simulink model "BPSK____TRANSMITTER"  (R2022a)
settings: Solver=VariableStepAuto  StartTime=0.0  StopTime=inf  RelTol=1e-3
values from neighbouring files (symbols this model uses):
  numSymsTot = length(message)    [generatemessage____BPSK.m]
undefined symbols (not defined in the file or in its folder): Fs, ip, usb
libraries: commfilt2 x2, dspsrcs4 x2, plutoradiolib x1, commdigbbndpm3 x1, simulink x1
settings Model: Creator=Nithish  LastModifiedBy=Nithish

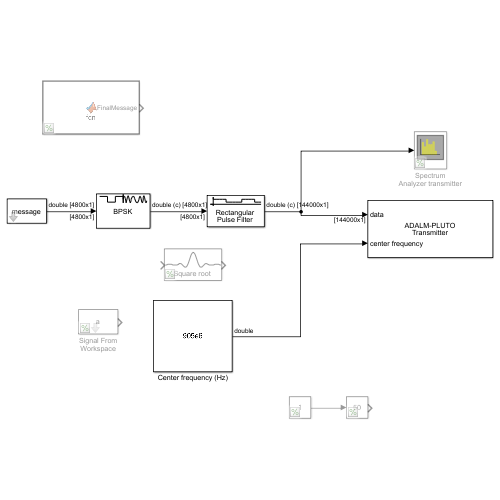
[thumbnail: Simulink's stored preview of the top-level diagram]
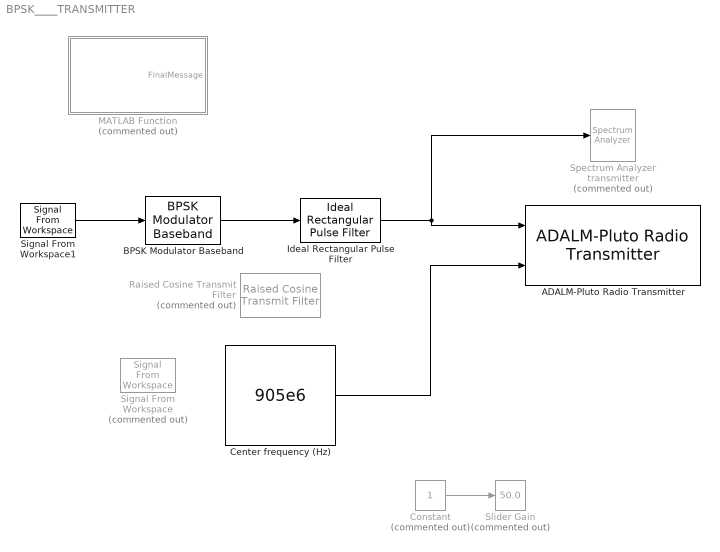
== system BPSK____TRANSMITTER ==
  ADALM-Pluto Radio Transmitter : plutoradiolib/ADALM-Pluto Radio Transmitter  RadioID=usb:0  uri=ip:10.0.0.200  CenterFrequencySource=Input Port  CenterFrequency=2.4e9  GainSource=Dialog  Gain=<binary blob, 139 chars, not shown>  ChannelMapping=1  BasebandSampleRate=240e3  UnderflowOutputPort=off  ShowAdvancedProperties=off  UseCustomFilter=off  filtPathRates=[737280000 11520000 3840000 1920000 960000 240000]  filtCoefficients=[-192 82 85 -215 228 -102 -110 290 -318 145 160 -426 471 -215 -238 633 -697 318 349 -923 1009 -457 -498 1309 -1423 640 693 -1812 1959 -876 -945 2458 -2647 1180 1268 -3290 3534 -1572 -1688 4375 -4698 2091 2247 -5836 6284 -2807 -3031 7918 -8588 3870 4225 -11182 12324 -5662 -6330 17255 -19735 9507 11312 -33568 43355 -25227 -42139 305542 305542 -42139 -25227 43355 -33568 11312 9507 -19735 17255 -6330 -5662 12324 -11182 4225 3870 -8588 7918 -3031 -2807 6284 -5836 2247 2091 -4698 4375 -1688 -1572 3534 -3290 1268 1180 -2647 2458 -945 -876 1959 -1812 693 640 -1423 1309 -498 -457 1009 -923 349 318 -697 633 -238 -215 471 -426 160 145 -318 290 -110 -102 228 -215 85 82 -192]  filtCoefficientSize=128  filtDecimInterpFactor=4  filtGain=-12  filtRFBandwidth=18000000  filterConfigStruct=struct()  DataSourceSelect=Input Port  DDSTone1Freq=5e3  DDSTone2Freq=10e3  DDSTone1Scale=0.5  DDSTone2Scale=0.25  DataTimeout=Inf  FrequencyCorrection=0  ENSMPinControlMode=None  BISTLoopbackMode=Disabled  BISTToneInject=Disabled  BISTSignalGen=PRBS  BISTToneFreq=Fs/32  BISTToneLevel=0
      settings: SourceProductBaseCode=PLUTO
  BPSK Modulator Baseband : commdigbbndpm3/BPSK Modulator Baseband  Ph=0  outDtype=double  outWordLen=16  outUDDataType=sfix(16)  outFracLenMode=Best precision  outFracLen=15  outDataTypeStr=double  outLastDataTypeStr=double
  Center frequency (Hz) : Constant  Value=905e6
  Constant : Constant  Commented=on
  Ideal Rectangular Pulse Filter : commfilt2/Ideal Rectangular Pulse Filter  pulseLen=30  pulseDelay=0  InputProcessing=Columns as channels (frame based)  RateOptions=Enforce single-rate processing  sampMode=Mute  normCheck=off  normMode=Sum of samples  filterGain=1  saveAsFlag=0  roundingMode=Floor  overflowMode=off  firstCoeffDataTypeStr=Inherit: Same word length as input  firstCoeffMin=[]  firstCoeffMax=[]  firstCoeffLastDataTypeStr=Inherit: Same word length as input  outputDataTypeStr=Inherit: Same as accumulator  outputMin=[]  outputMax=[]  outputLastDataTypeStr=Inherit: Same as accumulator
      settings: SourceProductBaseCode=CM
  MATLAB Function : MATLAB Function  Commented=on  TreatAsAtomicUnit=on
  Raised Cosine Transmit Filter : commfilt2/Raised Cosine Transmit Filter  Commented=on  filtType=Square root  R=0.5  filtSpan=4  N=10  filterGain=1  InputProcessing=Columns as channels (frame based)  RateOptions=Enforce single-rate processing  framing=Mute  checkCoeff=off  variableName=rcTxFilt  checkGain=Normalized  sampMode=Mute  saveAsFlag=0  currentFiltSpan=10  D=5  launchFVT=on  roundingMode=Floor  overflowMode=off  coeffDataTypeStr=Inherit: Same word length as input  coeffMin=[]  coeffMax=[]  coeffLastDataTypeStr=Inherit: Same word length as input  outputDataTypeStr=Inherit: Same as accumulator  outputMin=[]  outputMax=[]  outputLastDataTypeStr=Inherit: Same as accumulator
  Signal From Workspace : dspsrcs4/Signal From Workspace  Commented=on  X=a  Ts=1/8e3  nsamps=3000  OutputAfterFinalValue=Cyclic repetition  ignoreOrWarnInputAndFrameLengths=off  OutputFrames=off
  Signal From Workspace1 : dspsrcs4/Signal From Workspace  X=message  Ts=1/8e3  nsamps=numSymsTot*10  OutputAfterFinalValue=Cyclic repetition  ignoreOrWarnInputAndFrameLengths=off  OutputFrames=off
  Slider Gain : simulink/Math Operations/Slider Gain  Commented=on  gain=50.0  low=0  high=50
  Spectrum Analyzer transmitter : SpectrumAnalyzer  Commented=on
  wires:
  Ideal Rectangular Pulse Filter/1 -> ADALM-Pluto Radio Transmitter/1, Spectrum Analyzer transmitter/1
  Center frequency (Hz)/1 -> ADALM-Pluto Radio Transmitter/2
  BPSK Modulator Baseband/1 -> Ideal Rectangular Pulse Filter/1
  Constant/1 -> Slider Gain/1
  Signal From Workspace1/1 -> BPSK Modulator Baseband/1

== matlab function BPSK____TRANSMITTER/MATLAB Function ==
  data: FinalMessage output
function FinalMessage = fcn()
%% generateMessage.m

%clear all;
%close all;

%% Create message.
a = dec2bin('Hi Nithish. How are you? We are communicating from Mars.\n',8);
numChars = size(a,1);
fprintf(char(bin2dec(a)));

% this line converts binary strings into vectors
a = a - '0';

% reshape into a vector of bits; 8 bits per character
a = reshape(a.',8*numChars,1)';

% make sure string is properly recovered
b = reshape(a, 8, numChars).';
b = num2str(b);
fprintf(char(bin2dec(b)));

%% Build transmit packet
pre = [0 0 0 0 1 1 1 1 0 0 0 0 1 1 1 1];
message = [pre a];
numSymsTot = length(message);

j = 1;
FinalMessage = zeros(10*numSymsTot,1);
for i = 1:10*numSymsTot
   
    if j>numSymsTot
        j=1;
    end   
    
    FinalMessage(i) = message(j);
   
    j = j+1;
end
